simulink model "Target_Control_System"  (R2021b)
settings: Solver=FixedStepDiscrete  StartTime=0.0  StopTime=5  RelTol=1e-3
PreLoadFcn:
  | RTWConfigurationCB('preloadfcn', bdroot);
PostLoadFcn:
  | load('configuration/data_struct.mat');
  | load('configuration/fluxMaps_propMotor.mat');
  | load('configuration/parameterInit_PROP.mat');
  | load('configuration/parameterInit_PUMP.mat');
  | load('configuration/parameterInit_PITCH.mat');
  | load('configuration/parameterInit_TILT.mat');
  | %load('configuration/base_workspace_signal_definition.mat');
  | %load('resolvedatastores_to_baseworkspace_for_faster_simulation.mat');
model workspace (MAT data in the model file):
  SIMULATION_OPTIONS : Simulink.Parameter (value not decoded)
  TARGET_CODE_GEN : Simulink.Parameter (value not decoded)
  TCS_SAMPLE_FREQ_HZ : Simulink.Parameter (value not decoded)
symbols that are objects in the model workspace (value not decoded): TARGET_CODE_GEN, TCS_SAMPLE_FREQ_HZ
undefined symbols (not defined in the file): A_DQ_REF_LPF_INIT__PITCH, A_DQ_REF_LPF_INIT__PROP, A_DQ_REF_LPF_INIT__PUMP, A_DQ_REF_LPF_INIT__TILT, A_OBSERVER_CONFIDENCE_INIT__PITCH, A_OBSERVER_CONFIDENCE_INIT__PROP, A_OBSERVER_CONFIDENCE_INIT__PUMP, A_OBSERVER_CONFIDENCE_INIT__TILT, ACTUATOR_MAX_ANGLE_TRIP__PITCH, ACTUATOR_MIN_ANGLE_TRIP__PITCH, ACTUATOR_POS_SENSOR_INV_DIRECTION__PITCH, ACTUATOR_POS_SENSOR_INV_DIRECTION__TILT, ACTUATOR_POS_SENSOR_OFFSET__PITCH, ACTUATOR_POS_SENSOR_OFFSET__TILT, ADC_scaler1_baseaddr_TILT, ADC_SCALER_FLOAT_TO_FIXPOINT_EXPANSION, ANGLE_ELEC_FROM_SENSOR_OFFSET_INIT__PITCH, ANGLE_ELEC_FROM_SENSOR_OFFSET_INIT__PROP, ANGLE_ELEC_FROM_SENSOR_OFFSET_INIT__PUMP, ANGLE_ELEC_FROM_SENSOR_OFFSET_INIT__TILT, AUTO_CLEAR_FAULTS_ENABLED__PITCH, AUTO_CLEAR_FAULTS_ENABLED__PROP, AUTO_CLEAR_FAULTS_ENABLED__PUMP, AUTO_CLEAR_FAULTS_ENABLED__TILT, AUTO_CLEAR_FAULTS_WAIT_TICKS__PITCH, AUTO_CLEAR_FAULTS_WAIT_TICKS__PROP, AUTO_CLEAR_FAULTS_WAIT_TICKS__PUMP, AUTO_CLEAR_FAULTS_WAIT_TICKS__TILT, AUTO_I_ZERO_IDLE_TICKS__PITCH, AUTO_I_ZERO_IDLE_TICKS__PROP, AUTO_I_ZERO_IDLE_TICKS__PUMP, AUTO_I_ZERO_IDLE_TICKS__TILT, AUTO_I_ZERO_OFFSET_IDC_THRESHOLD__PITCH, AUTO_I_ZERO_OFFSET_IDC_THRESHOLD__PROP, AUTO_I_ZERO_OFFSET_IDC_THRESHOLD__PUMP, AUTO_I_ZERO_OFFSET_IDC_THRESHOLD__TILT, AUTO_I_ZERO_OFFSET_IPH_THRESHOLD__PITCH, AUTO_I_ZERO_OFFSET_IPH_THRESHOLD__PROP, AUTO_I_ZERO_OFFSET_IPH_THRESHOLD__PUMP, AUTO_I_ZERO_OFFSET_IPH_THRESHOLD__TILT, AUTO_SENSORLESS_SWITCHOVER_DISABLE_OMEGA, AUTO_SENSORLESS_SWITCHOVER_ENABLE_OMEGA, AUTO_SENSORLESS_SWITCHOVER_MIN_CONFIDENCE, AUXILIARY_PROTECTION_UNIT_BASEADDR__TILT, blanking_max_error_omega_INIT_PITCH, blanking_max_error_omega_INIT_TILT, blanking_max_error_position_INIT_PITCH, blanking_max_error_position_INIT_TILT, BRUTE_START_I_Q_REF_RAMP_SPEED__PITCH, BRUTE_START_I_Q_REF_RAMP_SPEED__PROP, BRUTE_START_I_Q_REF_RAMP_SPEED__PUMP, BRUTE_START_I_Q_REF_RAMP_SPEED__TILT, CONTROL_LOOP_DT_INIT__PITCH, CONTROL_LOOP_DT_INIT__PROP, CONTROL_LOOP_DT_INIT__PUMP, CONTROL_LOOP_DT_INIT__TILT, CORRECTION_FILTER_SCALE__PITCH, CORRECTION_FILTER_SCALE__PROP, CORRECTION_FILTER_SCALE__PUMP, CORRECTION_FILTER_SCALE__TILT ... (+458)
libraries: simulink x178, Reusables_Lib x24
(part 2 of 47)

== system Target_Control_System/Target_Control_System/MainLoop ==
  pitchMotor_mainLoop : Subsystem
  propMotor_mainLoop : Subsystem
  pumpMotor_mainLoop : Subsystem
  tiltMotor_mainLoop : Subsystem
  Vabc_pwm_ticks : Outport
  Vabc_pump_pwm_ticks : Outport  Port=2
  Out3 : Outport  Port=3
  Out4 : Outport  Port=4
  wires:
  pumpMotor_mainLoop/1(Vabc_pump_pwm_ticks) -> Vabc_pump_pwm_ticks/1  "pumpMotor_PWMticks"
  propMotor_mainLoop/1(Out1) -> Vabc_pwm_ticks/1  "propMotor_PWMticks"
  tiltMotor_mainLoop/1(Vabc_pump_pwm_ticks) -> Out4/1  "tiltMotor_PWMticks"
  pitchMotor_mainLoop/1(Vabc_pump_pwm_ticks) -> Out3/1  "pitchMotor_PWMticks"

== system Target_Control_System/Target_Control_System/ModelSource ==
  note: 1) Add Subsystem or Model blocks as valid variant choices.
      | 2) You cannot connect blocks at this level. At simulation, connectivity is automatically
      | determined, based on the active variant and port name matching.
  DoNotIncludeCustomCode : Subsystem  TreatAsAtomicUnit=on  VariantControl=TARGET_CODE_GEN == 0
  IncludeCustomCode : Subsystem  TreatAsAtomicUnit=on  VariantControl=(default)

== system Target_Control_System/Target_Control_System/Simulation Controls ==
  note: FPGA
  pitchMotor_simControls2 : Inport
  pitchMotor_simControls3 : Inport  Port=2
  pitchMotor_simControls : Inport  Port=3
  pitchMotor_simControls1 : Inport  Port=4
  fpgaFeedback : Inport  Port=5
  Enable : EnablePort
  Bus Selector17 : BusSelector  OutputSignals=tiltMotor_FPGAfeedback
  Bus Selector18 : BusSelector  OutputSignals=pitchMotor_FPGAfeedback
  Simulation Data Store Initialization : Subsystem  Priority=1  TreatAsAtomicUnit=on
  pitchMotor : Subsystem  Priority=10
  pitchMotor1 : Subsystem
  propMotor : Subsystem  Priority=10
  pumpMotor : Subsystem  Priority=10
  tiltMotor : Subsystem  Priority=10
  tiltMotor1 : Subsystem
  wires:
  fpgaFeedback/1 -> Bus Selector17/1, Bus Selector18/1
  Bus Selector17/1 -> tiltMotor1/1(tiltMotor_fpgaFeedback)  "<tiltMotor_FPGAfeedback>"
  Bus Selector18/1 -> pitchMotor1/1(pitchMotor_fpgaFeedback)  "<pitchMotor_FPGAfeedback>"
  pitchMotor_simControls3/1 -> pumpMotor/1(pitchMotor_simControls)  "pumpMotor_simControls"
  pitchMotor_simControls2/1 -> propMotor/1(propMotor_simControls)  "propMotor_simControls"
  pitchMotor_simControls/1 -> pitchMotor/1(pitchMotor_simControls)  "pitchMotor_simControls"
  pitchMotor_simControls1/1 -> tiltMotor/1(pitchMotor_simControls)  "tiltMotor_simControls"

== system Target_Control_System/Target_Control_System/System Start ==

== system Target_Control_System/Target_Control_System/DEBUG_Scopes/2Pi_Mod2 ==
  Iabc1 : Inport
  Constant : Constant  Value=pi  OutDataTypeStr=single  SampleTime=-1
  "Constant " : Constant  Value=pi  OutDataTypeStr=single  SampleTime=-1
  Math Function : Math  Operator=mod  SignedPower=on  SaturateOnIntegerOverflow=on
  Modulo Constant : Constant  Value=2*pi  OutDataTypeStr=single  SampleTime=-1
  Sum1 : Sum  Inputs=|++
  Sum2 : Sum  Inputs=|+-
  Out1 : Outport
  wires:
  Sum2/1 -> Out1/1
  Constant/1 -> Sum2/2
  Math Function/1 -> Sum2/1
  Sum1/1 -> Math Function/1
  Iabc1/1 -> Sum1/1
  "Constant "/1 -> Sum1/2
  Modulo Constant/1 -> Math Function/2

== system Target_Control_System/Target_Control_System/DEBUG_Scopes/IIR1 ==
  Input : Inport
  Constant : Constant  Value=CoefficientA  OutDataTypeStr=single  SampleTime=-1
  Constant1 : Constant  Value=CoefficientB  OutDataTypeStr=single  SampleTime=-1
  Product : Product  OutDataTypeStr=single  RndMeth=Zero
  Product1 : Product  RndMeth=Zero
  Sum : Sum  Inputs=|++  OutDataTypeStr=single
  Unit Delay : UnitDelay  SampleTime=-1  HasFrameUpgradeWarning=on
  Output : Outport
  wires:
  Sum/1 -> Unit Delay/1, Output/1
  Unit Delay/1 -> Product/1
  Constant1/1 -> Product1/2
  Constant/1 -> Product/2
  Product/1 -> Sum/1
  Product1/1 -> Sum/2
  Input/1 -> Product1/1

== system Target_Control_System/Target_Control_System/DEBUG_Scopes/IIR2 ==
  Input : Inport
  Constant : Constant  Value=CoefficientA  OutDataTypeStr=single  SampleTime=-1
  Constant1 : Constant  Value=CoefficientB  OutDataTypeStr=single  SampleTime=-1
  Product : Product  OutDataTypeStr=single  RndMeth=Zero
  Product1 : Product  RndMeth=Zero
  Sum : Sum  Inputs=|++  OutDataTypeStr=single
  Unit Delay : UnitDelay  SampleTime=-1  HasFrameUpgradeWarning=on
  Output : Outport
  wires:
  Sum/1 -> Unit Delay/1, Output/1
  Unit Delay/1 -> Product/1
  Constant1/1 -> Product1/2
  Constant/1 -> Product/2
  Product/1 -> Sum/1
  Product1/1 -> Sum/2
  Input/1 -> Product1/1

== system Target_Control_System/Target_Control_System/DEBUG_Scopes/Pitch Motor Debug ==
  In1 : Inport
  pitchMotor_PWMticks : Inport  Port=2
  Add2 : Sum  Inputs=-+
  Bus Creator2 : BusCreator  Inputs=3
  Data Store Read : DataStoreRead  DataStoreName=oPitch  DataStoreElements=oPitch.oMot_.oState_.oPosSensor_.fOmegaEFromSensor_  IndexOptions=Index vector (dialog)  Indices=1  OutputSizes=1
  Data Store Read1 : DataStoreRead  DataStoreName=oPitch  DataStoreElements=oPitch.oMot_.oState_.oRampDataPos_.fSetpoint_  IndexOptions=Index vector (dialog)  Indices=1  OutputSizes=1
  Data Store Read10 : DataStoreRead  DataStoreName=oPitch  DataStoreElements=oPitch.oMot_.oState_.oRampDataIdRef_.fSetpoint_  IndexOptions=Index vector (dialog)  Indices=1  OutputSizes=1
  Data Store Read{3,89,100,109} (4 alike) : DataStoreRead  DataStoreName=oPitch  DataStoreElements=oPitch.oIsr_.oIn_.oAdcData_.fIa_  IndexOptions=Index vector (dialog)  Indices=1  OutputSizes=1
  Data Store Read101 : DataStoreRead  DataStoreName=oPitch  DataStoreElements=oPitch.oIsr_.oIn_.oAdcData_.fIb_  IndexOptions=Index vector (dialog)  Indices=1  OutputSizes=1
  Data Store Read102 : DataStoreRead  DataStoreName=oPitch  DataStoreElements=oPitch.oIsr_.oIn_.oAdcData_.fIc_  IndexOptions=Index vector (dialog)  Indices=1  OutputSizes=1
  Data Store Read105 : DataStoreRead  DataStoreName=oPitch  DataStoreElements=oPitch.oMot_.oState_.oRampDataOmegaERef_.fRampOut_  IndexOptions=Index vector (dialog)  Indices=1  OutputSizes=1
  Data Store Read106 : DataStoreRead  DataStoreName=oPitch  DataStoreElements=oPitch.oMot_.oState_.oRampDataOmegaERef_.fSetpoint_  IndexOptions=Index vector (dialog)  Indices=1  OutputSizes=1
  Data Store Read107 : DataStoreRead  DataStoreName=oPitch  DataStoreElements=oPitch.oIsr_.oState_.fUdcPostlpf_  IndexOptions=Index vector (dialog)  Indices=1  OutputSizes=1
  Data Store Read108 : DataStoreRead  DataStoreName=oPitch  DataStoreElements=oPitch.oMot_.oState_.oRampDataIqRef_.fRampOut_  IndexOptions=Index vector (dialog)  Indices=1  OutputSizes=1
  Data Store Read11 : DataStoreRead  DataStoreName=oPitch  DataStoreElements=oPitch.oIsr_.oIn_.fIdRefRampOut_  IndexOptions=Index vector (dialog)  Indices=1  OutputSizes=1
  Data Store Read110 : DataStoreRead  DataStoreName=oPitch  DataStoreElements=oPitch.oMot_.oIn_.fIdSetpoint_  IndexOptions=Index vector (dialog)  Indices=1  OutputSizes=1
  Data Store Read12 : DataStoreRead  DataStoreName=oPitch  DataStoreElements=oPitch.oIsr_.oState_.fId_  IndexOptions=Index vector (dialog)  Indices=1  OutputSizes=1
  Data Store Read13 : DataStoreRead  DataStoreName=oPitch  DataStoreElements=oPitch.oMot_.oParam_.fUdcMaxTrip_  IndexOptions=Index vector (dialog)  Indices=1  OutputSizes=1
  Data Store Read14 : DataStoreRead  DataStoreName=oPitch  DataStoreElements=oPitch.oMot_.oParam_.fIdcMinTrip_  IndexOptions=Index vector (dialog)  Indices=1  OutputSizes=1
  Data Store Read15 : DataStoreRead  DataStoreName=oPitch  DataStoreElements=oPitch.oMot_.oParam_.fIdcMaxTrip_  IndexOptions=Index vector (dialog)  Indices=1  OutputSizes=1
  Data Store Read16 : DataStoreRead  DataStoreName=oPitch  DataStoreElements=oPitch.oIsr_.oIn_.fAngleElecFromPosSensor_  IndexOptions=Index vector (dialog)  Indices=1  OutputSizes=1
  Data Store Read17 : DataStoreRead  DataStoreName=oPitch  DataStoreElements=oPitch.oMot_.oParam_.fUdcMinTrip_  IndexOptions=Index vector (dialog)  Indices=1  OutputSizes=1
  Data Store Read18 : DataStoreRead  DataStoreName=oPitch  DataStoreElements=oPitch.oMot_.oOut_.fIdcLpf_  IndexOptions=Index vector (dialog)  Indices=1  OutputSizes=1
  Data Store Read19 : DataStoreRead  DataStoreName=oPitch  DataStoreElements=oPitch.oMot_.oParam_.fTripLimitSoftwareA_  IndexOptions=Index vector (dialog)  Indices=1  OutputSizes=1
  Data Store Read2 : DataStoreRead  DataStoreName=oPitch  DataStoreElements=oPitch.oMot_.oOut_.fUdcLpf_  IndexOptions=Index vector (dialog)  Indices=1  OutputSizes=1
  Data Store Read20 : DataStoreRead  DataStoreName=oPitch  DataStoreElements=oPitch.oMot_.oIn_.fIPhaseMagnitude_  IndexOptions=Index vector (dialog)  Indices=1  OutputSizes=1
  Data Store Read4 : DataStoreRead  DataStoreName=oPitch  DataStoreElements=oPitch.oMot_.oState_.uiDriveState_  IndexOptions=Index vector (dialog)  Indices=1  OutputSizes=1
  Data Store Read44 : DataStoreRead  DataStoreName=oPitch  DataStoreElements=oPitch.oMot_.oState_.oPosSensor_.oGbx_.fCurrentOutputAngle_  IndexOptions=Index vector (dialog)  Indices=1  OutputSizes=1
  Data Store Read5 : DataStoreRead  DataStoreName=oPitch  DataStoreElements=oPitch.oIsr_.oIn_.oAdcData_.fIb_  IndexOptions=Index vector (dialog)  Indices=1  OutputSizes=1
  Data Store Read6 : DataStoreRead  DataStoreName=oPitch  DataStoreElements=oPitch.oIsr_.oIn_.oAdcData_.fIc_  IndexOptions=Index vector (dialog)  Indices=1  OutputSizes=1
  Data Store Read7 : DataStoreRead  DataStoreName=oPitch  DataStoreElements=oPitch.oMot_.oState_.fIqRefBeforeRamp_  IndexOptions=Index vector (dialog)  Indices=1  OutputSizes=1
  Data Store Read72 : DataStoreRead  DataStoreName=oPitch  DataStoreElements=oPitch.oMot_.oState_.oRampDataPos_.fRampOut_  IndexOptions=Index vector (dialog)  Indices=1  OutputSizes=1
  Data Store Read8 : DataStoreRead  DataStoreName=oPitch  DataStoreElements=oPitch.oIsr_.oIn_.fIqRefRampOut_  IndexOptions=Index vector (dialog)  Indices=1  OutputSizes=1
  Data Store Read81 : DataStoreRead  DataStoreName=oPitch  DataStoreElements=oPitch.oIsr_.oState_.fId_  IndexOptions=Index vector (dialog)  Indices=1  OutputSizes=1
  Data Store Read82 : DataStoreRead  DataStoreName=oPitch  DataStoreElements=oPitch.oIsr_.oOut_.fTEstimate_  IndexOptions=Index vector (dialog)  Indices=1  OutputSizes=1
  Data Store Read83 : DataStoreRead  DataStoreName=oPitch  DataStoreElements=oPitch.oIsr_.oState_.fOmegaEObserverLpf2_  IndexOptions=Index vector (dialog)  Indices=1  OutputSizes=1
  Data Store Read84 : DataStoreRead  DataStoreName=oPitch  DataStoreElements=oPitch.oMot_.oState_.oRampDataIqRef_.fSetpoint_  IndexOptions=Index vector (dialog)  Indices=1  OutputSizes=1
  Data Store Read85 : DataStoreRead  DataStoreName=oPitch  DataStoreElements=oPitch.oIsr_.oState_.fIq_  IndexOptions=Index vector (dialog)  Indices=1  OutputSizes=1
  Data Store Read86 : DataStoreRead  DataStoreName=oPitch  DataStoreElements=oPitch.oMot_.oParam_.fPolePairs_  IndexOptions=Index vector (dialog)  Indices=1  OutputSizes=1
  Data Store Read87 : DataStoreRead  DataStoreName=oPitch  DataStoreElements=oPitch.oIsr_.oState_.fFluxMasterAngle_  IndexOptions=Index vector (dialog)  Indices=1  OutputSizes=1
  Data Store Read88 : DataStoreRead  DataStoreName=oPitch  DataStoreElements=oPitch.oIsr_.oState_.fFluxMainMagnitudeLpf_  IndexOptions=Index vector (dialog)  Indices=1  OutputSizes=1
  Data Store Read9 : DataStoreRead  DataStoreName=oPitch  DataStoreElements=oPitch.oIsr_.oState_.fIq_  IndexOptions=Index vector (dialog)  Indices=1  OutputSizes=1
  Data Store Read90 : DataStoreRead  DataStoreName=oPitch  DataStoreElements=oPitch.oIsr_.oIn_.oAdcData_.fIb_  IndexOptions=Index vector (dialog)  Indices=1  OutputSizes=1
  Data Store Read91 : DataStoreRead  DataStoreName=oPitch  DataStoreElements=oPitch.oIsr_.oIn_.oAdcData_.fIc_  IndexOptions=Index vector (dialog)  Indices=1  OutputSizes=1
  Data Store Read94 : DataStoreRead  DataStoreName=oPitch  DataStoreElements=oPitch.oMot_.oState_.fIqRefBeforeRamp_  IndexOptions=Index vector (dialog)  Indices=1  OutputSizes=1
  Data Store Read95 : DataStoreRead  DataStoreName=oPitch  DataStoreElements=oPitch.oIsr_.oIn_.fIqRefRampOut_  IndexOptions=Index vector (dialog)  Indices=1  OutputSizes=1
  Data Store Read96 : DataStoreRead  DataStoreName=oPitch  DataStoreElements=oPitch.oIsr_.oState_.fIq_  IndexOptions=Index vector (dialog)  Indices=1  OutputSizes=1
  Data Store Read99 : DataStoreRead  DataStoreName=oPitch  DataStoreElements=oPitch.oMot_.oState_.uiDriveState_  IndexOptions=Index vector (dialog)  Indices=1  OutputSizes=1
  Data Type Conversion{,11..12,14..15} (5 alike) : DataTypeConversion  OutDataTypeStr=single
  Fcn2 : Fcn  Expr=u/(2*pi)*60
  Gain6 : Gain
  Gain7 : Gain  Gain=POLE_PAIRS_INIT__PITCH
  Mux1 : Mux  Inputs=5
  Mux{2..5,20,22..23,25,27,29} (10 alike) : Mux  Inputs=3
  Mux24 : Mux  Inputs=2
  Mux26 : Mux  Inputs=2
  Mux31 : Mux
  One_Over3 : Fcn  Expr=1/u
  Output Bus Selector10 : BusSelector  OutputSignals=fMotorSensorSpeed_
  Output Bus Selector12 : BusSelector  Commented=on  OutputSignals=torque_pitch
  Output Bus Selector13 : BusSelector  OutputSignals=fMotorSensorSpeed_
  Output Bus Selector9 : BusSelector  OutputSignals=fMotorSensorSpeed_
  Pitch Debug 1 : Scope  NumInputPorts=7
  Pitch Debug 2 : Scope  NumInputPorts=5
  Pitch Debug Faults : Scope  NumInputPorts=9
  Product7 : Product
  Rad/s to RPM4 : Gain  Gain=60/2/pi  OutDataTypeStr=single
  Rad/s to RPM5 : Gain  Gain=60/2/pi  OutDataTypeStr=single
  Rate Transition{8..9,11..12} (4 alike) : RateTransition  Deterministic=off
  Scope10 : Scope  NumInputPorts=6
  torque_pitch : Constant  Value=0  OutDataTypeStr=single
  torque_pitch1 : Constant  Value=0  OutDataTypeStr=single
  wires:
  torque_pitch1/1 -> Data Type Conversion14/1  "<torque_pitch>"
  Data Store Read19/1 -> Mux1/5
  Data Store Read7/1 -> Mux2/1
  Data Store Read15/1 -> Mux5/1
  Data Store Read5/1 -> Mux1/2
  Data Store Read14/1 -> Mux5/3
  Mux2/1 -> Pitch Debug Faults/6
  Data Store Read18/1 -> Mux5/2
  Data Store Read12/1 -> Mux3/3
  Data Store Read4/1 -> Pitch Debug Faults/1
  Mux4/1 -> Pitch Debug Faults/2
  Data Store Read8/1 -> Mux2/2
  Data Store Read20/1 -> Mux1/4
  Data Store Read10/1 -> Mux3/1
  Data Store Read17/1 -> Mux4/3
  Mux1/1 -> Pitch Debug Faults/5
  Data Store Read13/1 -> Mux4/1
  Data Store Read11/1 -> Mux3/2
  Data Store Read9/1 -> Mux2/3
  Data Store Read2/1 -> Mux4/2
  Mux3/1 -> Pitch Debug Faults/7
  pitchMotor_PWMticks/1 -> Pitch Debug Faults/4
  Data Store Read6/1 -> Mux1/3
  Data Store Read3/1 -> Mux1/1
  Mux5/1 -> Pitch Debug Faults/3
  Mux20/1 -> Pitch Debug 2/5
  Data Store Read1/1 -> Mux20/1
  Data Store Read44/1 -> Mux20/3
  Data Store Read72/1 -> Mux20/2
  Data Type Conversion/1 -> Gain7/1
  Mux27/1 -> Pitch Debug 2/2
  In1/1 -> Output Bus Selector13/1, Output Bus Selector9/1, Output Bus Selector12/1, Output Bus Selector10/1
  Data Store Read106/1 -> Mux31/1
  Data Store Read101/1 -> Mux29/2
  Bus Creator2/1 -> Scope10/1
  Data Store Read100/1 -> Mux29/1
  One_Over3/1 -> Product7/2
  Mux24/1 -> Pitch Debug 1/1
  Rad/s to RPM4/1 -> Product7/1
  Data Store Read84/1 -> Mux23/1
  Data Type Conversion14/1 -> Mux26/1
  Rate Transition8/1 -> Scope10/6
  Data Type Conversion11/1 -> Scope10/4
  Data Store Read86/1 -> One_Over3/1
  Product7/1 -> Mux24/2
  Data Store Read110/1 -> Rate Transition12/1
  Data Store Read90/1 -> Mux25/2
  Data Store Read108/1 -> Rate Transition9/1
  Data Store Read109/1 -> Rate Transition11/1
  Data Type Conversion12/1 -> Mux24/1
  Mux26/1 -> Pitch Debug 1/6
  Fcn2/1 -> Scope10/3
  Data Store Read91/1 -> Mux25/3
  Data Store Read16/1 -> Mux22/1, Add2/2
  Data Store Read102/1 -> Mux29/3
  Data Store Read82/1 -> Mux26/2
  Rate Transition11/1 -> Bus Creator2/1
  Data Store Read107/1 -> Rate Transition8/1
  Data Store Read94/1 -> Mux27/1
  Data Store Read83/1 -> Rad/s to RPM4/1
  Data Store Read88/1 -> Pitch Debug 1/5
  Rate Transition12/1 -> Bus Creator2/3
  Output Bus Selector9/1 -> Rad/s to RPM5/1  "<fMotorSensorSpeed_>"
  Mux23/1 -> Pitch Debug 1/2
  Data Store Read95/1 -> Mux27/2
  Data Store Read85/1 -> Mux23/2
  Add2/1 -> Gain6/1
  Mux22/1 -> Pitch Debug 1/3
  Gain6/1 -> Mux22/3
  Data Store Read99/1 -> Pitch Debug 2/1
  Mux31/1 -> Pitch Debug 2/4
  Data Store Read105/1 -> Mux31/3
  Mux25/1 -> Pitch Debug 1/4
  Data Store Read/1 -> Mux31/2
  Data Store Read89/1 -> Mux25/1
  torque_pitch/1 -> Data Type Conversion11/1  "<torque_pitch>"
  Data Store Read96/1 -> Mux27/3
  Rad/s to RPM5/1 -> Data Type Conversion12/1
  Output Bus Selector13/1 -> Data Type Conversion/1  "<fMotorSensorSpeed_>"
  Output Bus Selector10/1 -> Data Type Conversion15/1  "<fMotorSensorSpeed_>"
  Data Type Conversion15/1 -> Fcn2/1
  Mux29/1 -> Pitch Debug 2/3
  Gain7/1 -> Mux31/4
  Rate Transition9/1 -> Bus Creator2/2
  Data Store Read87/1 -> Mux22/2, Add2/1
  Data Store Read81/1 -> Mux23/3

== system Target_Control_System/Target_Control_System/DEBUG_Scopes/Pump Motor Debug ==
  In1 : Inport
  2Pi_Mod1 : Subsystem
  2Pi_Mod2 : Subsystem  Commented=on
  Add1 : Sum  Inputs=-+
  Bus Creator1 : BusCreator  Inputs=3
  Constant3 : Constant  Value=1e-3  OutDataTypeStr=single  SampleTime=-1
  Constant4 : Constant  OutDataTypeStr=single  SampleTime=-1
  DC Link Voltage1 : Display
      settings: Format=decimal (Stored Integer)
  Data Store Read34 : DataStoreRead  DataStoreName=oPump  DataStoreElements=oPump.oIsr_.oState_.fUdcPostlpf_  IndexOptions=Index vector (dialog)  Indices=1  OutputSizes=1
  Data Store Read35 : DataStoreRead  DataStoreName=oPump  DataStoreElements=oPump.oMot_.oIn_.fIdSetpoint_  IndexOptions=Index vector (dialog)  Indices=1  OutputSizes=1
  Data Store Read36 : DataStoreRead  DataStoreName=oPump  DataStoreElements=oPump.oMot_.oState_.oRampDataIqRef_.fRampOut_  IndexOptions=Index vector (dialog)  Indices=1  OutputSizes=1
  Data Store Read37 : DataStoreRead  DataStoreName=oPump  DataStoreElements=oPump.oIsr_.oIn_.oAdcData_.fIdc_  IndexOptions=Index vector (dialog)  Indices=1  OutputSizes=1
  Data Store Read38 : DataStoreRead  DataStoreName=oPump  DataStoreElements=oPump.oIsr_.oState_.fUdcPostlpf_  IndexOptions=Index vector (dialog)  Indices=1  OutputSizes=1
  Data Store Read39 : DataStoreRead  DataStoreName=oPump  DataStoreElements=oPump.oMot_.oState_.fIdleCtrlOmegaEMin_  IndexOptions=Index vector (dialog)  Indices=1  OutputSizes=1
  Data Store Read40 : DataStoreRead  DataStoreName=oPump  DataStoreElements=oPump.oMot_.oState_.fIdleCtrlCurrent_  IndexOptions=Index vector (dialog)  Indices=1  OutputSizes=1
  Data Store Read41 : DataStoreRead  DataStoreName=oPump  DataStoreElements=oPump.oMot_.oState_.fIqRefBeforeRamp_  IndexOptions=Index vector (dialog)  Indices=1  OutputSizes=1
  Data Store Read43 : DataStoreRead  DataStoreName=oPump  DataStoreElements=oPump.oIsr_.oState_.fId_  IndexOptions=Index vector (dialog)  Indices=1  OutputSizes=1
  Data Store Read44 : DataStoreRead  DataStoreName=oPump  DataStoreElements=oPump.oIsr_.oState_.fFluxMasterAngle_  IndexOptions=Index vector (dialog)  Indices=1  OutputSizes=1
  Data Store Read45 : DataStoreRead  DataStoreName=oPump  DataStoreElements=oPump.oIsr_.oState_.fOmegaEObserverLpf2_  IndexOptions=Index vector (dialog)  Indices=1  OutputSizes=1
  Data Store Read46 : DataStoreRead  DataStoreName=oPump  DataStoreElements=oPump.oMot_.oState_.oRampDataIqRef_.fRampOut_  IndexOptions=Index vector (dialog)  Indices=1  OutputSizes=1
  Data Store Read47 : DataStoreRead  DataStoreName=oPump  DataStoreElements=oPump.oMot_.oState_.oRampDataIqRef_.fSetpoint_  IndexOptions=Index vector (dialog)  Indices=1  OutputSizes=1
  Data Store Read48 : DataStoreRead  DataStoreName=oPump  DataStoreElements=oPump.oIsr_.oState_.fIq_  IndexOptions=Index vector (dialog)  Indices=1  OutputSizes=1
  Data Store Read49 : DataStoreRead  DataStoreName=oPump  DataStoreElements=oPump.oMot_.oParam_.fPolePairs_  IndexOptions=Index vector (dialog)  Indices=1  OutputSizes=1
  Data Store Read50 : DataStoreRead  DataStoreName=oPump  DataStoreElements=oPump.oIsr_.oState_.fFluxMasterAngle_  IndexOptions=Index vector (dialog)  Indices=1  OutputSizes=1
  Data Store Read52 : DataStoreRead  DataStoreName=oPump  DataStoreElements=oPump.oIsr_.oIn_.fIqRefRampOut_  IndexOptions=Index vector (dialog)  Indices=1  OutputSizes=1
  Data Store Read54 : DataStoreRead  DataStoreName=oPump  DataStoreElements=oPump.oIsr_.oState_.fIq_  IndexOptions=Index vector (dialog)  Indices=1  OutputSizes=1
  Data Store Read55 : DataStoreRead  DataStoreName=oPump  DataStoreElements=oPump.oIsr_.oState_.fFluxMainMagnitudeLpf_  IndexOptions=Index vector (dialog)  Indices=1  OutputSizes=1
  Data Store Read56 : DataStoreRead  DataStoreName=oPump  DataStoreElements=oPump.oIsr_.oIn_.oAdcData_.fIa_  IndexOptions=Index vector (dialog)  Indices=1  OutputSizes=1
  Data Store Read57 : DataStoreRead  DataStoreName=oPump  DataStoreElements=oPump.oIsr_.oIn_.oAdcData_.fIb_  IndexOptions=Index vector (dialog)  Indices=1  OutputSizes=1
  Data Store Read58 : DataStoreRead  DataStoreName=oPump  DataStoreElements=oPump.oIsr_.oIn_.oAdcData_.fIc_  IndexOptions=Index vector (dialog)  Indices=1  OutputSizes=1
  Data Store Read60 : DataStoreRead  DataStoreName=oPump  DataStoreElements=oPump.oIsr_.oState_.fFluxMainAngleRaw2_  IndexOptions=Index vector (dialog)  Indices=1  OutputSizes=1
  Data Store Read61 : DataStoreRead  DataStoreName=oPump  DataStoreElements=oPump.oMot_.oState_.fIqRefBeforeRamp_  IndexOptions=Index vector (dialog)  Indices=1  OutputSizes=1
  Data Store Read62 : DataStoreRead  DataStoreName=oPump  DataStoreElements=oPump.oMot_.oParam_.fForcedAngleIRef_  IndexOptions=Index vector (dialog)  Indices=1  OutputSizes=1
  Data Store Read63 : DataStoreRead  DataStoreName=oPump  DataStoreElements=oPump.oMot_.oState_.oRampDataFluxMstrAngFrcd2clsdSmoothn_.fRampOut_  IndexOptions=Index vector (dialog)  Indices=1  OutputSizes=1
  Data Store Read64 : DataStoreRead  DataStoreName=oPump  DataStoreElements=oPump.oMot_.oState_.uiDriveState_  IndexOptions=Index vector (dialog)  Indices=1  OutputSizes=1
  Data Store Read65 : DataStoreRead  DataStoreName=oPump  DataStoreElements=oPump.oIsr_.oIn_.oAdcData_.fIa_  IndexOptions=Index vector (dialog)  Indices=1  OutputSizes=1
  Data Store Read70 : DataStoreRead  DataStoreName=oPump  DataStoreElements=oPump.oMot_.oIn_.fIdSetpoint_  IndexOptions=Index vector (dialog)  Indices=1  OutputSizes=1
  Data Store Read71 : DataStoreRead  DataStoreName=oPump  DataStoreElements=oPump.oIsr_.oIn_.oAdcData_.fIa_  IndexOptions=Index vector (dialog)  Indices=1  OutputSizes=1
  Data Store Read72 : DataStoreRead  DataStoreName=oPump  DataStoreElements=oPump.oIsr_.oIn_.oAdcData_.fIb_  IndexOptions=Index vector (dialog)  Indices=1  OutputSizes=1
  Data Store Read73 : DataStoreRead  DataStoreName=oPump  DataStoreElements=oPump.oIsr_.oState_.fUdcPostlpf_  IndexOptions=Index vector (dialog)  Indices=1  OutputSizes=1
  Data Store Read74 : DataStoreRead  DataStoreName=oPump  DataStoreElements=oPump.oIsr_.oIn_.oAdcData_.fIc_  IndexOptions=Index vector (dialog)  Indices=1  OutputSizes=1
  Data Store Read75 : DataStoreRead  DataStoreName=oPump  DataStoreElements=oPump.oMot_.oParam_.fForcedAngleOmegaEHandoff_  IndexOptions=Index vector (dialog)  Indices=1  OutputSizes=1
  Data Store Read76 : DataStoreRead  DataStoreName=oPump  DataStoreElements=oPump.oMot_.oState_.oRampDataOmegaERef_.fRampOut_  IndexOptions=Index vector (dialog)  Indices=1  OutputSizes=1
  Data Store Read77 : DataStoreRead  DataStoreName=oPump  DataStoreElements=oPump.oMot_.oState_.oRampDataOmegaERef_.fRampOut_  IndexOptions=Index vector (dialog)  Indices=1  OutputSizes=1
  Data Store Read80 : DataStoreRead  DataStoreName=oPump  DataStoreElements=oPump.oMot_.oState_.oRampDataOmegaERef_.fSetpoint_  IndexOptions=Index vector (dialog)  Indices=1  OutputSizes=1
  Data Type Conversion10 : DataTypeConversion  Commented=on  OutDataTypeStr=single
  Data Type Conversion7 : DataTypeConversion  OutDataTypeStr=single
  Data Type Conversion8 : DataTypeConversion  OutDataTypeStr=single
  Data Type Conversion9 : DataTypeConversion  OutDataTypeStr=single
  Divide1 : Product  Inputs=*/
  Efficiency1 : Display
      settings: Format=decimal (Stored Integer)
  Fcn1 : Fcn  Expr=u/(2*pi)*60
  Gain3 : Gain
  Gain4 : Gain  Gain=1/POLE_PAIRS_INIT__PUMP
  Gain5 : Gain  Gain=POLE_PAIRS_INIT__PUMP
  IIR3 : Subsystem  mask{CoefficientA=0.7, CoefficientB=0.3}
      mask prompts: CoefficientA "First Coefficient (long)"; CoefficientB "Second Coefficient (short)"
  IIR4 : Subsystem  mask{CoefficientA=0.7, CoefficientB=0.3}
      mask prompts: CoefficientA "First Coefficient (long)"; CoefficientB "Second Coefficient (short)"
  IdRef1 : Display
      settings: Format=decimal (Stored Integer)
  Inverter Input Power1 : Display
      settings: Format=decimal (Stored Integer)
  IqRef1 : Display
      settings: Format=decimal (Stored Integer)
  Mux10 : Mux  Inputs=2
  Mux{12..15,17..18,20..21} (8 alike) : Mux  Inputs=3
  Mux16 : Mux  Inputs=2
  Mux19 : Mux  Inputs=2
  One_Over2 : Fcn  Expr=1/u
  Output Bus Selector4 : BusSelector  Commented=on  OutputSignals=position_electrical_pump
  Output Bus Selector5 : BusSelector  OutputSignals=fMotorSensorSpeed_
  Output Bus Selector6 : BusSelector  OutputSignals=fMotorSensorSpeed_
  Output Bus Selector7 : BusSelector  OutputSignals=fMotorSensorSpeed_
  PP1 : Gain  Commented=on  Gain=POLE_PAIRS_INIT__PUMP  OutDataTypeStr=single
  Product4 : Product  Inputs=3
  Product5 : Product
  Product6 : Product
  Pump Debug 1 : Scope  NumInputPorts=7
  Pump Debug 2 : Scope  NumInputPorts=7
  Rad/s to RPM2 : Gain  Gain=60/2/pi  OutDataTypeStr=single
  Rad/s to RPM3 : Gain  Gain=60/2/pi  OutDataTypeStr=single
  Rate Transition{1..4,7} (5 alike) : RateTransition  Deterministic=off
  Scope5 : Scope
  Scope6 : Scope  NumInputPorts=6
  Shaft Power (kW)1 : Display
      settings: Format=decimal (Stored Integer)
  Speed (RPM)1 : Display
      settings: Format=decimal (Stored Integer)
  Subtract2 : Sum  Inputs=+-
  Subtract3 : Sum  Inputs=+-
  Torque & Speed to kW1 : Gain  Gain=1/9.5488*1e-3
  Torque (Nm)1 : Display
      settings: Format=decimal (Stored Integer)
  position_pump : Constant  Value=0  OutDataTypeStr=single
  pump_torque : Constant  Value=0  OutDataTypeStr=single
  wires:
  position_pump/1 -> 2Pi_Mod1/1(Iabc1)
  Data Store Read73/1 -> DC Link Voltage1/1
  Data Store Read57/1 -> Mux20/2
  Data Store Read76/1 -> Mux16/2
  Constant4/1 -> Subtract3/1
  Data Store Read64/1 -> Pump Debug 2/1
  Data Type Conversion7/1 -> Mux10/2, Fcn1/1
  [pump_fRpmActual] -> Speed (RPM)1/1
  Subtract2/1 -> Divide1/1
  Bus Creator1/1 -> Scope6/1
  Data Store Read58/1 -> Mux20/3
  Data Store Read37/1 -> IIR4/1(Input)
  Data Store Read48/1 -> Mux18/2
  IIR4/1(Output) -> Product4/1
  Mux10/1 -> Scope5/1
  Data Store Read47/1 -> Mux18/1
  Gain4/1 -> Mux10/1
  Output Bus Selector6/1 -> Data Type Conversion7/1  "<fMotorSensorSpeed_>"
  Data Store Read40/1 -> Mux14/2
  Data Store Read75/1 -> Mux16/1
  Mux16/1 -> Pump Debug 2/5
  Product4/1 -> Inverter Input Power1/1, Subtract2/1
  Torque & Speed to kW1/1 -> Scope6/5, Subtract2/2, Divide1/2, Shaft Power (kW)1/1  "ShaftPower"
  Data Store Read46/1 -> Rate Transition2/1
  Mux20/1 -> Pump Debug 1/4
  Data Store Read61/1 -> Mux14/3  "fIdleCtrlCurrent_"
  Mux18/1 -> Pump Debug 1/2
  Add1/1 -> Gain3/1
  Data Store Read62/1 -> Mux14/1
  Data Store Read60/1 -> Mux21/2
  PP1/1 -> 2Pi_Mod2/1(Iabc1)
  Data Type Conversion8/1 -> Scope6/4, Torque (Nm)1/1, Product5/2
  Data Store Read41/1 -> Mux12/1
  Mux19/1 -> Pump Debug 1/1
  ? -> Data Type Conversion10/1
  Data Store Read49/1 -> One_Over2/1
  Data Store Read63/1 -> Mux21/3
  Data Store Read70/1 -> Rate Transition4/1
  Data Store Read77/1 -> Mux17/3
  Data Store Read74/1 -> Mux15/3
  Data Store Read52/1 -> Mux12/2
  Rate Transition7/1 -> Gain4/1
  Subtract3/1 -> Efficiency1/1
  Rad/s to RPM3/1 -> Data Type Conversion9/1
  One_Over2/1 -> Product6/2
  Fcn1/1 -> Scope6/3, Product5/1, [pump_fRpmActual]
  Data Store Read43/1 -> Mux18/3
  Rate Transition3/1 -> Bus Creator1/1
  Output Bus Selector7/1 -> Rad/s to RPM3/1  "<fMotorSensorSpeed_>"
  Data Store Read71/1 -> Mux15/1
  Rate Transition2/1 -> Bus Creator1/2
  Data Store Read44/1 -> Mux21/1
  Mux21/1 -> Pump Debug 1/6
  IIR3/1(Output) -> Product4/2
  Mux15/1 -> Pump Debug 2/4
  Divide1/1 -> Subtract3/2
  [Sensorless_Omega] -> Rate Transition7/1
  Data Store Read34/1 -> Rate Transition1/1
  Data Store Read55/1 -> Pump Debug 1/5
  Product5/1 -> Torque & Speed to kW1/1
  Mux13/1 -> Pump Debug 1/3
  Data Store Read80/1 -> Mux17/1
  Data Store Read36/1 -> IqRef1/1
  Mux17/1 -> Pump Debug 2/6
  Gain3/1 -> Mux13/3
  Gain5/1 -> Pump Debug 2/7
  In1/1 -> Output Bus Selector6/1, Output Bus Selector5/1, Output Bus Selector7/1, Output Bus Selector4/1
  Output Bus Selector5/1 -> Gain5/1  "<fMotorSensorSpeed_>"
  Data Store Read39/1 -> Mux17/2
  Data Store Read45/1 -> Rad/s to RPM2/1
  Constant3/1 -> Product4/3
  Data Type Conversion9/1 -> Mux19/1
  Data Store Read38/1 -> IIR3/1(Input)
  Data Store Read65/1 -> Rate Transition3/1
  Rate Transition1/1 -> Scope6/6
  pump_torque/1 -> Data Type Conversion8/1  "<torque_pump>"
  Data Store Read54/1 -> Mux12/3
  Data Store Read56/1 -> Mux20/1
  Data Store Read35/1 -> IdRef1/1
  2Pi_Mod1/1(Out1) -> Mux13/1, Add1/2
  Data Type Conversion10/1 -> PP1/1
  Rad/s to RPM2/1 -> Product6/1
  Product6/1 -> Mux19/2
  Mux14/1 -> Pump Debug 2/2
  Data Store Read72/1 -> Mux15/2
  Rate Transition4/1 -> Bus Creator1/3
  Data Store Read50/1 -> Mux13/2, Add1/1
  Mux12/1 -> Pump Debug 2/3

== system Target_Control_System/Target_Control_System/DEBUG_Scopes/Tilt Motor Debug ==
  In1 : Inport
  Add2 : Sum  Inputs=-+
  Bus Creator2 : BusCreator  Inputs=3
  Data Store Read : DataStoreRead  DataStoreName=oTilt  DataStoreElements=oTilt.oMot_.oState_.oPosSensor_.fOmegaEFromSensor_  IndexOptions=Index vector (dialog)  Indices=1  OutputSizes=1
  Data Store Read1 : DataStoreRead  DataStoreName=oTilt  DataStoreElements=oTilt.oMot_.oState_.oRampDataPos_.fSetpoint_  IndexOptions=Index vector (dialog)  Indices=1  OutputSizes=1
  Data Store Read100 : DataStoreRead  DataStoreName=oTilt  DataStoreElements=oTilt.oIsr_.oIn_.oAdcData_.fIa_  IndexOptions=Index vector (dialog)  Indices=1  OutputSizes=1
  Data Store Read101 : DataStoreRead  DataStoreName=oTilt  DataStoreElements=oTilt.oIsr_.oIn_.oAdcData_.fIb_  IndexOptions=Index vector (dialog)  Indices=1  OutputSizes=1
  Data Store Read102 : DataStoreRead  DataStoreName=oTilt  DataStoreElements=oTilt.oIsr_.oIn_.oAdcData_.fIc_  IndexOptions=Index vector (dialog)  Indices=1  OutputSizes=1
  Data Store Read105 : DataStoreRead  DataStoreName=oTilt  DataStoreElements=oTilt.oMot_.oState_.oRampDataOmegaERef_.fRampOut_  IndexOptions=Index vector (dialog)  Indices=1  OutputSizes=1
  Data Store Read106 : DataStoreRead  DataStoreName=oTilt  DataStoreElements=oTilt.oMot_.oState_.oRampDataOmegaERef_.fSetpoint_  IndexOptions=Index vector (dialog)  Indices=1  OutputSizes=1
  Data Store Read107 : DataStoreRead  DataStoreName=oTilt  DataStoreElements=oTilt.oIsr_.oState_.fUdcPostlpf_  IndexOptions=Index vector (dialog)  Indices=1  OutputSizes=1
  Data Store Read108 : DataStoreRead  DataStoreName=oTilt  DataStoreElements=oTilt.oMot_.oState_.oRampDataIqRef_.fRampOut_  IndexOptions=Index vector (dialog)  Indices=1  OutputSizes=1
  Data Store Read109 : DataStoreRead  DataStoreName=oTilt  DataStoreElements=oTilt.oIsr_.oIn_.oAdcData_.fIa_  IndexOptions=Index vector (dialog)  Indices=1  OutputSizes=1
  Data Store Read110 : DataStoreRead  DataStoreName=oTilt  DataStoreElements=oTilt.oMot_.oIn_.fIdSetpoint_  IndexOptions=Index vector (dialog)  Indices=1  OutputSizes=1
  Data Store Read16 : DataStoreRead  DataStoreName=oTilt  DataStoreElements=oTilt.oIsr_.oIn_.fAngleElecFromPosSensor_  IndexOptions=Index vector (dialog)  Indices=1  OutputSizes=1
  Data Store Read44 : DataStoreRead  DataStoreName=oTilt  DataStoreElements=oTilt.oMot_.oState_.oPosSensor_.oGbx_.fCurrentOutputAngle_  IndexOptions=Index vector (dialog)  Indices=1  OutputSizes=1
  Data Store Read72 : DataStoreRead  DataStoreName=oTilt  DataStoreElements=oTilt.oMot_.oState_.oRampDataPos_.fRampOut_  IndexOptions=Index vector (dialog)  Indices=1  OutputSizes=1
  Data Store Read81 : DataStoreRead  DataStoreName=oTilt  DataStoreElements=oTilt.oIsr_.oState_.fId_  IndexOptions=Index vector (dialog)  Indices=1  OutputSizes=1
  Data Store Read82 : DataStoreRead  DataStoreName=oTilt  DataStoreElements=oTilt.oIsr_.oOut_.fTEstimate_  IndexOptions=Index vector (dialog)  Indices=1  OutputSizes=1
  Data Store Read83 : DataStoreRead  DataStoreName=oTilt  DataStoreElements=oTilt.oIsr_.oState_.fOmegaEObserverLpf2_  IndexOptions=Index vector (dialog)  Indices=1  OutputSizes=1
  Data Store Read84 : DataStoreRead  DataStoreName=oTilt  DataStoreElements=oTilt.oMot_.oState_.oRampDataIqRef_.fSetpoint_  IndexOptions=Index vector (dialog)  Indices=1  OutputSizes=1
  Data Store Read85 : DataStoreRead  DataStoreName=oTilt  DataStoreElements=oTilt.oIsr_.oState_.fIq_  IndexOptions=Index vector (dialog)  Indices=1  OutputSizes=1
  Data Store Read86 : DataStoreRead  DataStoreName=oTilt  DataStoreElements=oTilt.oMot_.oParam_.fPolePairs_  IndexOptions=Index vector (dialog)  Indices=1  OutputSizes=1
  Data Store Read87 : DataStoreRead  DataStoreName=oTilt  DataStoreElements=oTilt.oIsr_.oState_.fFluxMasterAngle_  IndexOptions=Index vector (dialog)  Indices=1  OutputSizes=1
  Data Store Read88 : DataStoreRead  DataStoreName=oTilt  DataStoreElements=oTilt.oIsr_.oState_.fFluxMainMagnitudeLpf_  IndexOptions=Index vector (dialog)  Indices=1  OutputSizes=1
  Data Store Read89 : DataStoreRead  DataStoreName=oTilt  DataStoreElements=oTilt.oIsr_.oIn_.oAdcData_.fIa_  IndexOptions=Index vector (dialog)  Indices=1  OutputSizes=1
  Data Store Read90 : DataStoreRead  DataStoreName=oTilt  DataStoreElements=oTilt.oIsr_.oIn_.oAdcData_.fIb_  IndexOptions=Index vector (dialog)  Indices=1  OutputSizes=1
  Data Store Read91 : DataStoreRead  DataStoreName=oTilt  DataStoreElements=oTilt.oIsr_.oIn_.oAdcData_.fIc_  IndexOptions=Index vector (dialog)  Indices=1  OutputSizes=1
  Data Store Read94 : DataStoreRead  DataStoreName=oTilt  DataStoreElements=oTilt.oMot_.oState_.fIqRefBeforeRamp_  IndexOptions=Index vector (dialog)  Indices=1  OutputSizes=1
  Data Store Read95 : DataStoreRead  DataStoreName=oTilt  DataStoreElements=oTilt.oIsr_.oIn_.fIqRefRampOut_  IndexOptions=Index vector (dialog)  Indices=1  OutputSizes=1
  Data Store Read96 : DataStoreRead  DataStoreName=oTilt  DataStoreElements=oTilt.oIsr_.oState_.fIq_  IndexOptions=Index vector (dialog)  Indices=1  OutputSizes=1
  Data Store Read99 : DataStoreRead  DataStoreName=oTilt  DataStoreElements=oTilt.oMot_.oState_.uiDriveState_  IndexOptions=Index vector (dialog)  Indices=1  OutputSizes=1
  Data Type Conversion{,11..12,14..15} (5 alike) : DataTypeConversion  OutDataTypeStr=single
  Fcn2 : Fcn  Expr=u/(2*pi)*60
  Gain6 : Gain
  Gain7 : Gain  Gain=POLE_PAIRS_INIT__TILT
  Mux{20,22..23,25,27,29} (6 alike) : Mux  Inputs=3
  Mux24 : Mux  Inputs=2
  Mux26 : Mux  Inputs=2
  Mux31 : Mux
  One_Over3 : Fcn  Expr=1/u
  Output Bus Selector10 : BusSelector  OutputSignals=fMotorSensorSpeed_
  Output Bus Selector12 : BusSelector  Commented=on  OutputSignals=torque_tilt
  Output Bus Selector13 : BusSelector  OutputSignals=fMotorSensorSpeed_
  Output Bus Selector9 : BusSelector  OutputSignals=fMotorSensorSpeed_
  Product7 : Product
  Rad/s to RPM4 : Gain  Gain=60/2/pi  OutDataTypeStr=single
  Rad/s to RPM5 : Gain  Gain=60/2/pi  OutDataTypeStr=single
  Rate Transition{8..9,11..12} (4 alike) : RateTransition  Deterministic=off
  Scope10 : Scope  NumInputPorts=6
  Tilt Debug 1 : Scope  NumInputPorts=7
  Tilt Debug 2 : Scope  NumInputPorts=5
  torque_tilt : Constant  Value=0  OutDataTypeStr=single
  torque_tilt1 : Constant  Value=0  OutDataTypeStr=single
  wires:
  torque_tilt1/1 -> Data Type Conversion14/1  "<torque_tilt>"
  Mux20/1 -> Tilt Debug 2/5
  Data Store Read1/1 -> Mux20/1
  Data Store Read44/1 -> Mux20/3
  Data Store Read72/1 -> Mux20/2
  Data Type Conversion/1 -> Gain7/1
  Mux27/1 -> Tilt Debug 2/2
  In1/1 -> Output Bus Selector13/1, Output Bus Selector9/1, Output Bus Selector12/1, Output Bus Selector10/1  "motorMeasure_tilt"
  Data Store Read106/1 -> Mux31/1
  Data Store Read101/1 -> Mux29/2
  Bus Creator2/1 -> Scope10/1
  Data Store Read100/1 -> Mux29/1
  One_Over3/1 -> Product7/2
  Mux24/1 -> Tilt Debug 1/1
  Rad/s to RPM4/1 -> Product7/1
  Data Store Read84/1 -> Mux23/1
  Data Type Conversion14/1 -> Mux26/1
  Rate Transition8/1 -> Scope10/6
  Data Type Conversion11/1 -> Scope10/4
  Data Store Read86/1 -> One_Over3/1
  Product7/1 -> Mux24/2
  Data Store Read110/1 -> Rate Transition12/1
  Data Store Read90/1 -> Mux25/2
  Data Store Read108/1 -> Rate Transition9/1
  Data Store Read109/1 -> Rate Transition11/1
  Data Type Conversion12/1 -> Mux24/1
  Mux26/1 -> Tilt Debug 1/6
  Fcn2/1 -> Scope10/3
  Output Bus Selector12/1 -> ?  "<torque_tilt>"
  Data Store Read91/1 -> Mux25/3
  Data Store Read16/1 -> Mux22/1, Add2/2
  Data Store Read102/1 -> Mux29/3
  Data Store Read82/1 -> Mux26/2
  Rate Transition11/1 -> Bus Creator2/1
  Data Store Read107/1 -> Rate Transition8/1
  Data Store Read94/1 -> Mux27/1
  Data Store Read83/1 -> Rad/s to RPM4/1
  Data Store Read88/1 -> Tilt Debug 1/5
  Rate Transition12/1 -> Bus Creator2/3
  Output Bus Selector9/1 -> Rad/s to RPM5/1  "<fMotorSensorSpeed_>"
  Mux23/1 -> Tilt Debug 1/2
  Data Store Read95/1 -> Mux27/2
  Data Store Read85/1 -> Mux23/2
  Add2/1 -> Gain6/1
  Mux22/1 -> Tilt Debug 1/3
  Gain6/1 -> Mux22/3
  Data Store Read99/1 -> Tilt Debug 2/1
  Mux31/1 -> Tilt Debug 2/4
  Data Store Read105/1 -> Mux31/3
  Mux25/1 -> Tilt Debug 1/4
  Data Store Read/1 -> Mux31/2
  Data Store Read89/1 -> Mux25/1
  torque_tilt/1 -> Data Type Conversion11/1  "<torque_tilt>"
  Data Store Read96/1 -> Mux27/3
  Rad/s to RPM5/1 -> Data Type Conversion12/1
  Output Bus Selector13/1 -> Data Type Conversion/1  "<fMotorSensorSpeed_>"
  Output Bus Selector10/1 -> Data Type Conversion15/1  "<fMotorSensorSpeed_>"
  Data Type Conversion15/1 -> Fcn2/1
  Mux29/1 -> Tilt Debug 2/3
  Gain7/1 -> Mux31/4
  Rate Transition9/1 -> Bus Creator2/2
  Data Store Read87/1 -> Mux22/2, Add2/1
  Data Store Read81/1 -> Mux23/3

== system Target_Control_System/Target_Control_System/InterruptFunction/allMotors_readAdc ==
  PropMotorAdcFeedback : Inport  OutDataTypeStr=Bus: SAdcDataSingleIn_t
  PumpMotorAdcFeedback : Inport  Port=2  OutDataTypeStr=Bus: SAdcDataSingleIn_t
  PitchMotorAdcFeedback : Inport  Port=3  OutDataTypeStr=Bus: SAdcDataSingleIn_t
  TiltMotorAdcFeedback : Inport  Port=4  OutDataTypeStr=Bus: SAdcDataSingleIn_t
  adcDataToIsr : TriggerPort  TriggerType=function-call  VariantControl=(inherit)
  Code Gen Switch2 : Constant  Value=TARGET_CODE_GEN==1  OutDataTypeStr=boolean  SampleTime=-1
  Constant{1..4} (4 alike) : Constant  Value=TARGET_CODE_GEN~=1  OutDataTypeStr=boolean  SampleTime=-1
  Sensor Offset Calibration VP : Stateflow chart  TreatAsAtomicUnit=on
  codeGen_adcRead : Subsystem  TreatAsAtomicUnit=on
  pitchMotor_adcRead : Subsystem
  powerCalculations : Subsystem
  propMotor_adcRead : Subsystem
  pumpMotor_adcRead : Subsystem
  tiltMotor_adcRead : Subsystem
  wires:
  Code Gen Switch2/1 -> codeGen_adcRead/Enable
  TiltMotorAdcFeedback/1 -> tiltMotor_adcRead/1(TiltMotorAdcFeedback)
  Constant4/1 -> tiltMotor_adcRead/Enable
  PitchMotorAdcFeedback/1 -> pitchMotor_adcRead/1(PitchMotorAdcFeedback)
  Constant3/1 -> pitchMotor_adcRead/Enable
  PumpMotorAdcFeedback/1 -> pumpMotor_adcRead/1(PumpMotorAdcFeedback)
  Constant2/1 -> pumpMotor_adcRead/Enable
  Constant1/1 -> propMotor_adcRead/Enable
  PropMotorAdcFeedback/1 -> propMotor_adcRead/1(PropMotorAdcFeedback)
